simulink model "parte4_eje1_Thidraulica_ctrlV13"  (Simulink 8.1)
settings: Solver=ode45  SolverMode=SingleTasking  StartTime=0.0  StopTime=20  RelTol=1e-3
settings Model: Creator=cjuar  LastModifiedBy=cjuar  CovMetricSettings=dwe  CovHtmlReporting=off  covSaveCumulativeToWorkspaceVar=off  CovSaveSingleToWorkspaceVar=off  CovExternalEMLEnable=on
settings DataIOCC: LimitDataPoints=off  SaveFormat=StructureWithTime  SignalLoggingSaveFormat=Dataset
settings OptimizationCC: ExpressionDepthLimit=128
settings DebuggingCC: UnderspecifiedInitializationDetection=Simplified  MergeDetectMultiDrivingBlocksExec=error  SolverPrmCheckMsg=none  FcnCallInpInsideContextMsg=EnableAllAsError  FrameProcessingCompatibilityMsg=error  StateNameClashWarn=none  SFUnexpectedBacktrackingDiag=error  SFNoUnconditionalDefaultTransitionDiag=error
settings HardwareCC: ProdBitPerPointer=64  ProdLargestAtomicFloat=Float  ProdIntDivRoundTo=Zero  ProdEndianess=LittleEndian  ProdHWDeviceType=Specified
settings ModelReferenceCC: PropagateSignalLabelsOutOfModel=on
settings GRTTargetCC: CodeReplacementLibrary=C99 (ISO)  GeneratePreprocessorConditionals=Use local settings  CombineOutputUpdateFcns=on  GRTInterface=off

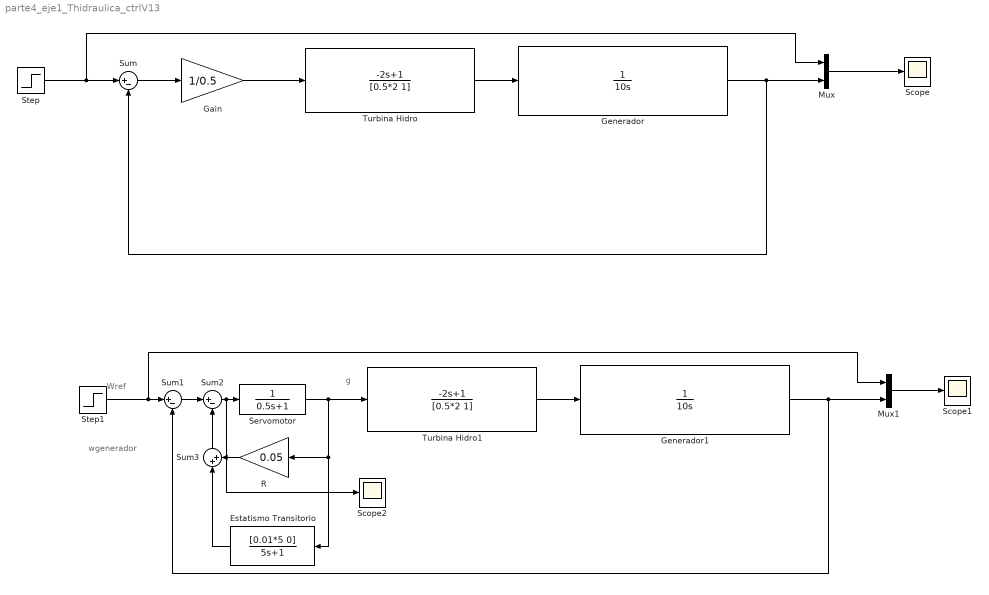
== system parte4_eje1_Thidraulica_ctrlV13 ==
  note: g
  note: wgenerador
  note: Wref
  Estatismo Transitorio : TransferFcn  Numerator=[0.01*5 0]  Denominator=[5 1]
  Gain : Gain  Gain=1/0.5
  Generador : TransferFcn  Denominator=[10 0]
  Generador1 : TransferFcn  Denominator=[10 0]
  Mux : Mux  Inputs=2
  Mux1 : Mux  Inputs=2
  R : Gain  Gain=0.05
  Scope : Scope
      settings: TimeRange=auto  MaxDataPoints=5000  SaveToWorkspace=off  SaveName=ScopeData  YMin=-0.03703  YMax=0.12309  SampleTime=-1
  Scope1 : Scope
      settings: TimeRange=auto  MaxDataPoints=5000  SaveToWorkspace=off  YMin=-0.02133  YMax=0.11348  SampleTime=-1
  Scope2 : Scope
      settings: TimeRange=auto  MaxDataPoints=5000  SaveToWorkspace=off  SaveName=ScopeData2  YMin=-0.01278  YMax=0.11501  SampleTime=-1
  Servomotor : TransferFcn  Denominator=[0.5 1]
  Step : Step  After=0.1  SampleTime=0
  Step1 : Step  After=0.1  SampleTime=0
  Sum : Sum  Inputs=|+-
  Sum1 : Sum  Inputs=|+-
  Sum2 : Sum  Inputs=|+-
  Sum3 : Sum  Inputs=|++
  Turbina Hidro : TransferFcn  Numerator=[-2 1]  Denominator=[0.5*2 1]
  Turbina Hidro1 : TransferFcn  Numerator=[-2 1]  Denominator=[0.5*2 1]
  wires:
  Mux/1 -> Scope/1
  Turbina Hidro/1 -> Generador/1
  Gain/1 -> Turbina Hidro/1
  Sum/1 -> Gain/1
  Generador/1 -> Sum/2, Mux/2
  Step/1 -> Mux/1, Sum/1
  Step1/1 -> Mux1/1, Sum1/1
  Mux1/1 -> Scope1/1
  Sum1/1 -> Sum2/1
  Generador1/1 -> Sum1/2, Mux1/2
  Turbina Hidro1/1 -> Generador1/1
  Sum3/1 -> Sum2/2
  R/1 -> Sum3/2
  Servomotor/1 -> Estatismo Transitorio/1, R/1, Turbina Hidro1/1
  Sum2/1 -> Scope2/1, Servomotor/1
  Estatismo Transitorio/1 -> Sum3/1
